simulink model "controller"  (R2020b)
settings: Solver=VariableStepAuto  StartTime=0.0  StopTime=100  MaxStep=0.01  RelTol=1e-3
values from neighbouring files (symbols this model uses):
  k_p = 0.1    [params.m]
  k_v = 0.5    [params.m]
  m = 1    [params.m]
  x_des = 6    [params.m]
settings Model: Creator=Danil  LastModifiedBy=Danil

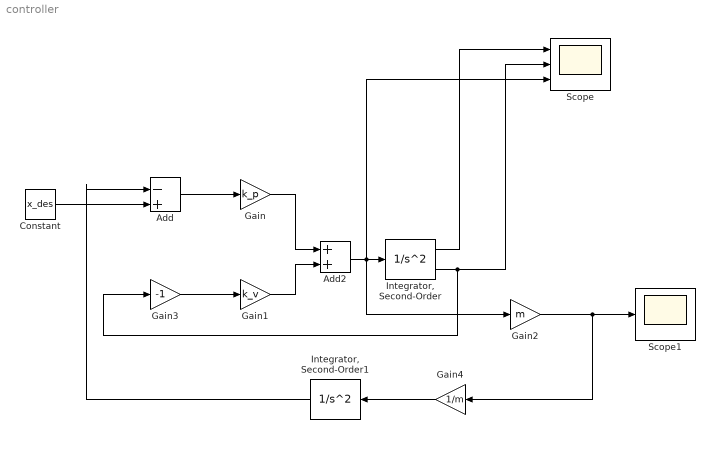
== system controller ==
  Add : Sum  Inputs=-|+
  Add2 : Sum
  Constant : Constant  Value=x_des
  Gain : Gain  Gain=k_p
  Gain1 : Gain  Gain=k_v
  Gain2 : Gain  Gain=m
  Gain3 : Gain  Gain=-1
  Gain4 : Gain  Gain=1/m
  "Integrator, Second-Order" : SecondOrderIntegrator
  "Integrator, Second-Order1" : SecondOrderIntegrator  ShowOutput=x
  Scope : Scope  NumInputPorts=3
  Scope1 : Scope
  wires:
  Add/1 -> Gain/1
  "Integrator, Second-Order"/1 -> Scope/1
  "Integrator, Second-Order"/2 -> Gain3/1, Scope/2
  Gain3/1 -> Gain1/1
  Gain/1 -> Add2/1
  Gain1/1 -> Add2/2
  Constant/1 -> Add/2
  Add2/1 -> Gain2/1, Scope/3, "Integrator, Second-Order"/1
  Gain2/1 -> Gain4/1, Scope1/1
  Gain4/1 -> "Integrator, Second-Order1"/1
  "Integrator, Second-Order1"/1 -> Add/1
